simulink model "setpoint_firefly"  (R2016a)
settings: Solver=FixedStepAuto  StartTime=0.0  StopTime=inf  FixedStep=0.05  RelTol=1e-3
undefined symbols (not defined in the file): Pose
libraries: robotlib x3
settings Model: Creator=ttpl4  LastModifiedBy=UNIST
settings OptimizationCC: OptimizeModelRefInitCode=on  LifeSpan=Inf  MaxStackSize=64
settings HardwareCC: ProdBitPerPointer=32  ProdLargestAtomicFloat=None  ProdIntDivRoundTo=Undefined  ProdEndianess=Unspecified  ProdWordSize=32  ProdHWDeviceType=Generic->Unspecified (assume 32-bit Generic)
settings RTWCC: SystemTargetFile=ert.tlc  HardwareBoard=Robot Operating System (ROS)  TemplateMakefile=ert_default_tmf  GenerateReport=on  Toolchain=Catkin  IncludeHyperlinkInReport=on  LaunchReport=on  TargetLang=C++  GenerateTraceInfo=on  GenerateTraceReport=on  GenerateTraceReportSl=on  GenerateTraceReportSf=on  GenerateTraceReportEml=on
settings CodeAppCC: ForceParamTrailComments=on  IgnoreCustomStorageClasses=off  OperatorAnnotations=on  SimulinkDataObjDesc=on  SFDataObjDesc=on  MATLABFcnDesc=on  InsertBlockDesc=on  MATLABSourceComments=on

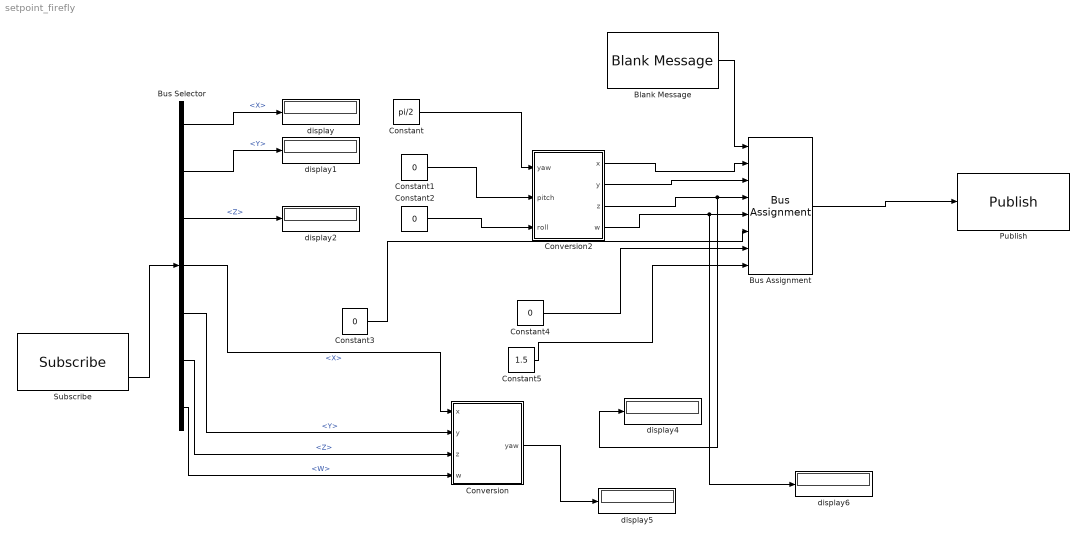
== system setpoint_firefly ==
  Blank Message : robotlib/Blank Message  SourceLibraryInfo=This block requires Robotics System Toolbox  messageType=geometry_msgs/PoseStamped  SampleTime=-1
  Bus Assignment : BusAssignment  AssignedSignals=Pose.Orientation.X,Pose.Orientation.Y,Pose.Orientation.Z,Pose.Orientation.W,Pose.Position.X,Pose.Position.Y,Pose.Position.Z
  Bus Selector : BusSelector  OutputSignals=Pose.Position.X,Pose.Position.Y,Pose.Position.Z,Pose.Orientation.X,Pose.Orientation.Y,Pose.Orientation.Z,Pose.Orientation.W
  Constant : Constant  Value=pi/2
  Constant{1..4} (4 alike) : Constant  Value=0
  Constant5 : Constant  Value=1.5
  Conversion : MATLAB Function  TreatAsAtomicUnit=on
  Conversion2 : MATLAB Function  TreatAsAtomicUnit=on
  Publish : robotlib/Publish  SourceLibraryInfo=This block requires Robotics System Toolbox  topicSource=Select from ROS network  topic=/mavros/setpoint_position/local  messageType=geometry_msgs/PoseStamped  messageQueueLength=1
  Subscribe : robotlib/Subscribe  SourceLibraryInfo=This block requires Robotics System Toolbox  topicSource=Select from ROS network  topic=/mavros/local_position/pose  messageType=geometry_msgs/PoseStamped  sampleTime=-1  messageQueueLength=1
  display{,1..2,4..6} (6 alike) : Display
  wires:
  Blank Message/1 -> Bus Assignment/1
  Bus Assignment/1 -> Publish/1
  Conversion2/4(w) -> display6/1, Bus Assignment/5
  Conversion2/3(z) -> display4/1, Bus Assignment/4
  Conversion2/2(y) -> Bus Assignment/3
  Conversion2/1(x) -> Bus Assignment/2
  Constant2/1 -> Conversion2/3(roll)
  Constant1/1 -> Conversion2/2(pitch)
  Constant/1 -> Conversion2/1(yaw)
  Constant3/1 -> Bus Assignment/6
  Constant4/1 -> Bus Assignment/7
  Constant5/1 -> Bus Assignment/8
  Subscribe/2 -> Bus Selector/1
  Bus Selector/1 -> display/1  "<X>"
  Bus Selector/2 -> display1/1  "<Y>"
  Bus Selector/3 -> display2/1  "<Z>"
  Bus Selector/4 -> Conversion/1(x)  "<X>"
  Bus Selector/5 -> Conversion/2(y)  "<Y>"
  Bus Selector/6 -> Conversion/3(z)  "<Z>"
  Conversion/1(yaw) -> display5/1
  Bus Selector/7 -> Conversion/4(w)  "<W>"

== matlab function setpoint_firefly/Conversion ==
  data: yaw output; x input; y input; z input; w input
function yaw  = quat2eul(x,y,z,w)
%#codegen

% Convert the quaternion to a yaw angle (zyx euler angle)
eul = quat2eul([w,x,y,z]);
yaw = eul(1);

end

== matlab function setpoint_firefly/Conversion2 ==
  data: yaw input; pitch input; roll input; x output; y output; z output; w output
function [x,   y,   z,   w]   = eul2quat(yaw,pitch,roll)
%#codegen

% Convert the quaternion to a yaw angle (zyx euler angle)
q = eul2quat([yaw,pitch,roll]);
w=q(1);
x=q(2);
y=q(3);
z=q(4);
end
